simulink model "target"  (R2016a)
settings: Solver=ode4  StartTime=0.0  StopTime=10.0  FixedStep=0.001  RelTol=1e-3
values from neighbouring files (symbols this model uses):
  g = 9.8    [initialization.m]
settings Model: Creator=asus  LastModifiedBy=asus

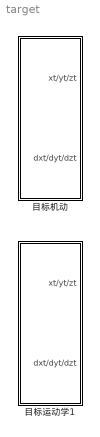
== system target ==
  目标机动 : Subsystem
  目标运动学1 : Subsystem

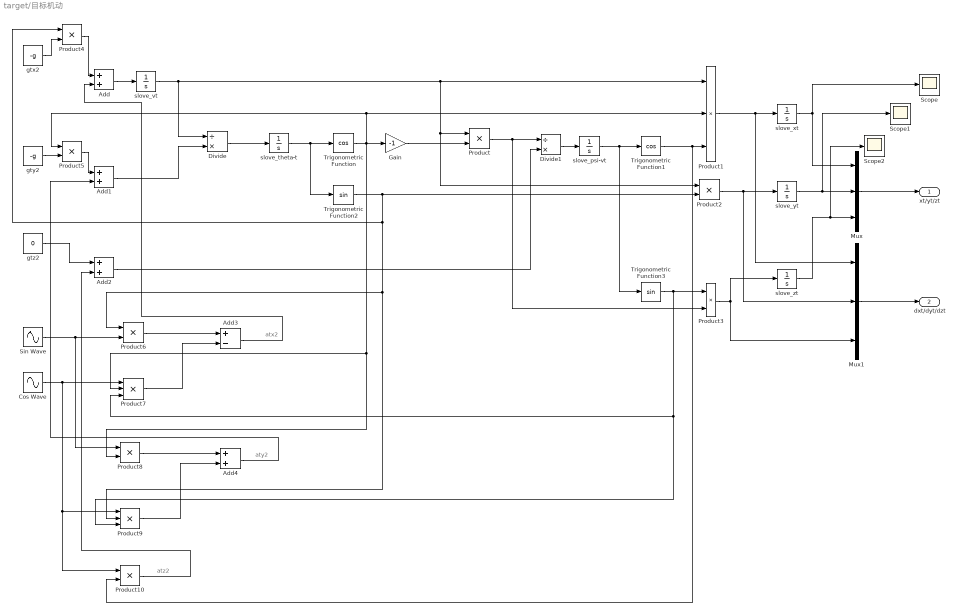
== system target/目标机动 ==
  note: atz2
  note: aty2
  note: atx2
  Add{,1..2,4} (4 alike) : Sum
  Add3 : Sum  Inputs=+-
  Cos Wave : Sin  Amplitude=7*9.8  Phase=pi/2  SampleTime=0
  Divide : Product  Inputs=/*
  Divide1 : Product  Inputs=/*
  Gain : Gain  Gain=-1
  Mux : Mux  Inputs=3
  Mux1 : Mux  Inputs=3
  Product{,2..6,8,10} (8 alike) : Product
  Product1 : Product  Inputs=3
  Product7 : Product  Inputs=3
  Product9 : Product  Inputs=3
  Scope : Scope
  Scope1 : Scope
  Scope2 : Scope
  Sin Wave : Sin  Amplitude=7*9.8  SampleTime=0
  Trigonometric Function : Trigonometry  Operator=cos
  Trigonometric Function1 : Trigonometry  Operator=cos
  Trigonometric Function2 : Trigonometry
  Trigonometric Function3 : Trigonometry
  gtx2 : Constant  Value=-g
  gty2 : Constant  Value=-g
  gtz2 : Constant  Value=0
  slove_psi-vt : Integrator  InitialCondition=120/57.3
  slove_theta-t : Integrator  InitialCondition=-30/57.3
  slove_vt : Integrator  InitialCondition=800
  slove_xt : Integrator  InitialCondition=11136
  slove_yt : Integrator  InitialCondition=8603.6
  slove_zt : Integrator  InitialCondition=5192.8
  xt/yt/zt : Outport
  dxt/dyt/dzt : Outport  Port=2
  wires:
  Trigonometric Function2/1 -> Product9/2, Product6/1, Product4/1, Product2/2
  Product2/1 -> Mux1/2, slove_yt/1
  Trigonometric Function3/1 -> Product9/3, Product7/3, Product3/1
  Trigonometric Function1/1 -> Product10/2, Product1/3
  Product3/1 -> Mux1/3, slove_zt/1
  Mux/1 -> xt/yt/zt/1
  Product1/1 -> Mux1/1, slove_xt/1
  gtz2/1 -> Add2/1
  Add2/1 -> Divide1/2
  Divide/1 -> slove_theta-t/1
  slove_zt/1 -> Scope2/1, Mux/3
  Product/1 -> Product3/2, Divide1/1
  slove_vt/1 -> Product2/1, Product/1, Product1/1, Divide/1
  slove_theta-t/1 -> Trigonometric Function2/1, Trigonometric Function/1
  Add/1 -> slove_vt/1
  Add1/1 -> Divide/2
  slove_xt/1 -> Scope/1, Mux/1
  Trigonometric Function/1 -> Product8/2, Product7/2, Product5/1, Product1/2, Gain/1
  Divide1/1 -> slove_psi-vt/1
  Gain/1 -> Product/2
  slove_psi-vt/1 -> Trigonometric Function3/1, Trigonometric Function1/1
  slove_yt/1 -> Scope1/1, Mux/2
  Mux1/1 -> dxt/dyt/dzt/1
  gtx2/1 -> Product4/2
  Product4/1 -> Add/1
  gty2/1 -> Product5/2
  Product5/1 -> Add1/1
  Product10/1 -> Add2/2
  Add4/1 -> Add1/2
  Sin Wave/1 -> Product8/1, Product6/2
  Cos Wave/1 -> Product10/1, Product9/1, Product7/1
  Product6/1 -> Add3/1
  Product7/1 -> Add3/2
  Add3/1 -> Add/2
  Product8/1 -> Add4/1
  Product9/1 -> Add4/2

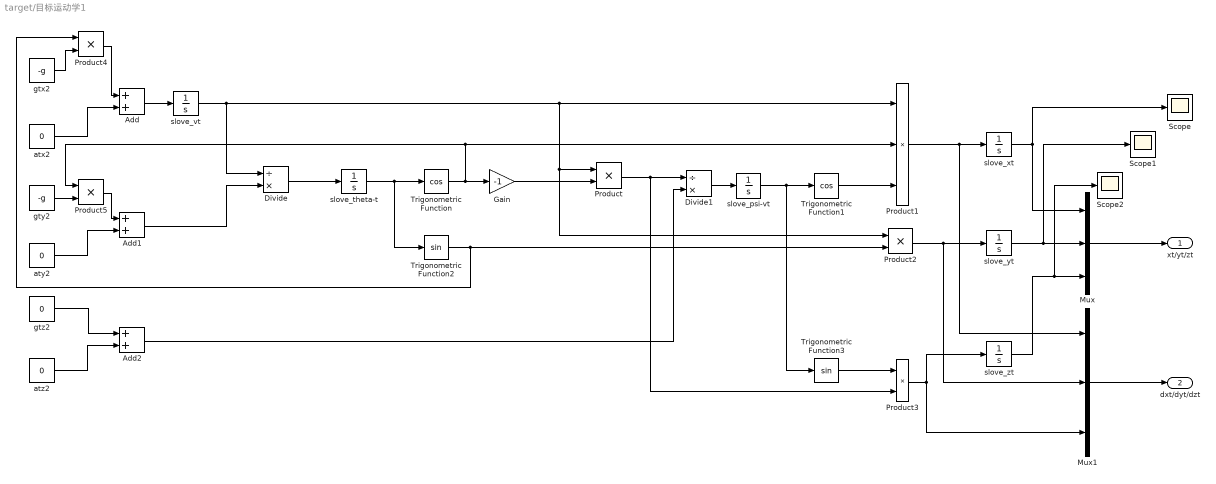
== system target/目标运动学1 ==
  Add : Sum
  Add1 : Sum
  Add2 : Sum
  Divide : Product  Inputs=/*
  Divide1 : Product  Inputs=/*
  Gain : Gain  Gain=-1
  Mux : Mux  Inputs=3
  Mux1 : Mux  Inputs=3
  Product{,2..5} (5 alike) : Product
  Product1 : Product  Inputs=3
  Scope : Scope
  Scope1 : Scope
  Scope2 : Scope
  Trigonometric Function : Trigonometry  Operator=cos
  Trigonometric Function1 : Trigonometry  Operator=cos
  Trigonometric Function2 : Trigonometry
  Trigonometric Function3 : Trigonometry
  atx2 : Constant  Value=0
  aty2 : Constant  Value=0
  atz2 : Constant  Value=0
  gtx2 : Constant  Value=-g
  gty2 : Constant  Value=-g
  gtz2 : Constant  Value=0
  slove_psi-vt : Integrator  InitialCondition=120/57.3
  slove_theta-t : Integrator  InitialCondition=-30/57.3
  slove_vt : Integrator  InitialCondition=800
  slove_xt : Integrator  InitialCondition=11136
  slove_yt : Integrator  InitialCondition=8603.6
  slove_zt : Integrator  InitialCondition=5192.8
  xt/yt/zt : Outport
  dxt/dyt/dzt : Outport  Port=2
  wires:
  Trigonometric Function2/1 -> Product4/1, Product2/2
  Product2/1 -> Mux1/2, slove_yt/1
  Trigonometric Function3/1 -> Product3/1
  Trigonometric Function1/1 -> Product1/3
  Product3/1 -> Mux1/3, slove_zt/1
  Mux/1 -> xt/yt/zt/1
  Product1/1 -> Mux1/1, slove_xt/1
  gtz2/1 -> Add2/1
  Add2/1 -> Divide1/2
  Divide/1 -> slove_theta-t/1
  aty2/1 -> Add1/2
  atz2/1 -> Add2/2
  slove_zt/1 -> Scope2/1, Mux/3
  Product/1 -> Product3/2, Divide1/1
  atx2/1 -> Add/2
  slove_vt/1 -> Product2/1, Product/1, Product1/1, Divide/1
  slove_theta-t/1 -> Trigonometric Function2/1, Trigonometric Function/1
  Add/1 -> slove_vt/1
  Add1/1 -> Divide/2
  slove_xt/1 -> Scope/1, Mux/1
  Trigonometric Function/1 -> Product5/1, Product1/2, Gain/1
  Divide1/1 -> slove_psi-vt/1
  Gain/1 -> Product/2
  slove_psi-vt/1 -> Trigonometric Function3/1, Trigonometric Function1/1
  slove_yt/1 -> Scope1/1, Mux/2
  Mux1/1 -> dxt/dyt/dzt/1
  gtx2/1 -> Product4/2
  Product4/1 -> Add/1
  gty2/1 -> Product5/2
  Product5/1 -> Add1/1
